simulink model "dvfs_zed_simple_backup"  (R2025b)
settings: Solver=FixedStepDiscrete  StartTime=0.0  StopTime=10.0  FixedStep=0.1  RelTol=1e-3
settings Model: Creator=Vimal Rency  LastModifiedBy=Vimal Rency

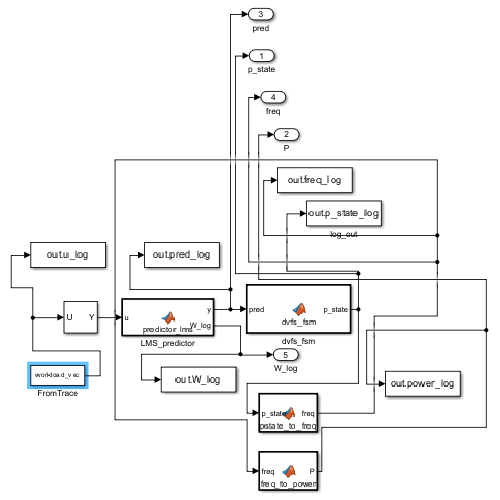
[thumbnail: Simulink's stored preview of the top-level diagram]
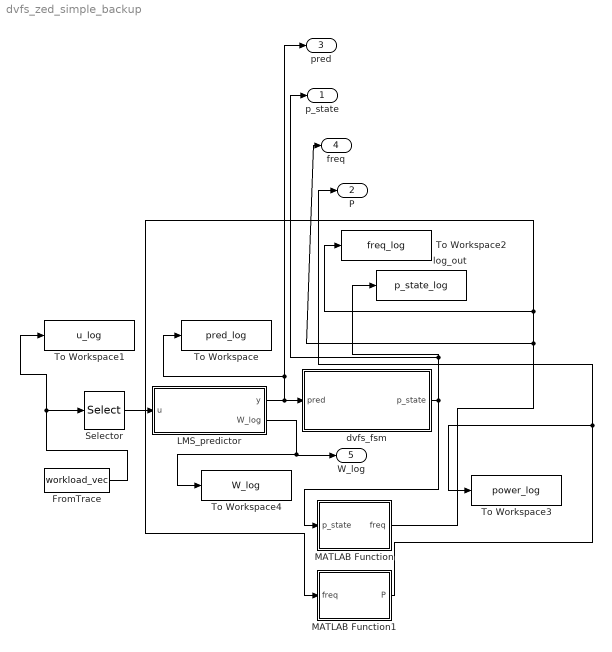
== system dvfs_zed_simple_backup ==
  FromTrace : FromWorkspace  VariableName=workload_vec
  LMS_predictor : MATLAB Function  TreatAsAtomicUnit=on
  MATLAB Function : MATLAB Function  TreatAsAtomicUnit=on
  MATLAB Function1 : MATLAB Function  TreatAsAtomicUnit=on
  Selector : Selector  NumberOfDimensions=2  InputPortWidth=3  IndexOptions=Select all,Index vector (dialog)  Indices=[1 3],1  OutputSizes=1,1
  To Workspace : ToWorkspace  VariableName=pred_log  SampleTime=-1
  To Workspace1 : ToWorkspace  VariableName=u_log  SampleTime=-1
  To Workspace2 : ToWorkspace  VariableName=freq_log  SampleTime=-1
  To Workspace3 : ToWorkspace  VariableName=power_log  SampleTime=-1
  To Workspace4 : ToWorkspace  VariableName=W_log  SampleTime=-1
  dvfs_fsm : MATLAB Function  TreatAsAtomicUnit=on
  log_out : ToWorkspace  VariableName=p_state_log  SampleTime=-1
  p_state : Outport
  P : Outport  Port=2
  pred : Outport  Port=3
  freq : Outport  Port=4
  W_log : Outport  Port=5
  wires:
  FromTrace/1 -> To Workspace1/1, Selector/1
  dvfs_fsm/1(p_state) -> MATLAB Function/1(p_state), log_out/1, p_state/1
  MATLAB Function1/1(P) -> P/1, To Workspace3/1
  MATLAB Function/1(freq) -> MATLAB Function1/1(freq), To Workspace2/1, freq/1
  LMS_predictor/1(y) -> dvfs_fsm/1(pred), pred/1, To Workspace/1
  LMS_predictor/2(W_log) -> W_log/1, To Workspace4/1
  Selector/1 -> LMS_predictor/1(u)

== matlab function dvfs_zed_simple_backup/LMS_predictor ==
  data: u input; y output; W_log output
function [y, W_log] = predictor_lms(u)
% Adaptive LMS Predictor
% u = current workload
% y = predicted next workload

persistent W mu prev
if isempty(W)
    W = 0.9;      % initial weight
    mu = 0.04;    % learning rate
    prev = 0.0;   % previous input
end

% Predict next workload
y = W * prev+0.02;

% LMS error
e = u - y;

% LMS weight update rule
W = W + mu * e * prev;

% Next iteration input
prev = u;

% Clamp output to [0–1]
y = max(0, min(1, y));
W_log = W;    
end

== matlab function dvfs_zed_simple_backup/MATLAB Function ==
  data: p_state input; freq output
function freq = pstate_to_freq(p_state)

switch p_state
    case 0
        freq = 100;   % MHz
    case 1
        freq = 200;
    case 2
        freq = 300;
    otherwise
        freq = 0;
end

end

== matlab function dvfs_zed_simple_backup/MATLAB Function1 ==
  data: freq input; P output
function P = freq_to_power(freq)

% simple model: Power ∝ frequency
P = 0.01 * freq;   % scale as you want (mW)

end

== matlab function dvfs_zed_simple_backup/dvfs_fsm ==
  data: pred input; p_state output
function p_state = dvfs_fsm(pred)
% 0=LOW, 1=MED, 2=HIGH

persistent state last_change cycle_cnt next_avail
if isempty(state)
    state = uint8(1); % start in MED
    last_change = uint32(0);
    cycle_cnt = uint32(0);
    next_avail = uint32(0);
end

cycle_cnt = cycle_cnt + 1;

T1 = 0.08;
T2 = 0.26;
H  = 0.02;
min_residency = uint32(0);
transition_latency = uint32(0);

desired = state;

switch state
    case uint8(0)        % LOW
        if pred >= T1 + H
            desired = uint8(1);
        end
    case uint8(1)        % MED
        if pred >= T2 + H
            desired = uint8(2);
        elseif pred < T1 - H
            desired = uint8(0);
        end
    case uint8(2)        % HIGH
        if pred < T2 - H
            desired = uint8(1);
        end
end

if desired ~= state
    state = desired;
    last_change = cycle_cnt;
    next_avail = cycle_cnt;
end


p_state = state;
end
